simulink model "Load_Flow_Simulink"  (R2020b)
settings: Solver=FixedStepDiscrete  StartTime=0.0  StopTime=inf  FixedStep=0.001  RelTol=1e-3  EnableMultiTasking=on
InitFcn:
  | s1_define_network
  | s2_network_setup
  | s4_ybus2
  | 
  | %s3_ybus1
  | %s4_ybus2
  | 
  | 
  | %s5_dummy_load
  | 
  | %load('loadsDummy.mat')
values from neighbouring files (symbols this model uses):
  ABI = availableBusIndices    [Create_Ybus.m]
  Admittance = zeros(numBranch*3,5*3)    [s4_ybus2.m]    (also in s4_ybus3.m)
  BusFromTo = [busFrom busTo]    [s2_network_setup.m]
  busIDs = str2double(busNames)    [s1_define_network.m]
  busNames = [busNames(1:substationIndex-1); busNames(substationIndex+1:end);                busNames(substationIndex)]    [s1_define_network.m]    (also in s2_network_setup.m = int16(str2num(cell2mat(busNames))); s4_ybus3.m = int16(str2num(cell2mat(busNames))); s5_dummy_load.m = int16(str2num(cell2mat(busNames))))
  Ibase = Vbase/Zbase    [s1_define_network.m]
  LineCodes = [lineCodes;2]    [s1_define_network.m]    (also in s2_network_setup.m = zeros(37,1))
  loadsDummy = [600 600 2000 3000 100 100 100 0 0 0 0 0 ... (42 elements, 7x6)]    [loadsDummy.mat]    (also in s1_define_network.m = loadsIn)
  MBI = missingBusIndices    [Create_Ybus.m]    (also in s2_network_setup.m = 0)
  N = numBus-1    [Create_Ybus.m]
  noLoadQuantities = v2struct(v0mags,v0phases,v0,w,wCheck,w3phase)    [Compute_No_Load_Voltage.m]    (also in s2_network_setup.m = Compute_No_Load_Voltage(Y,Y_NS,N,                           )
  numBranch = length(lineBuses1)    [Create_Ybus.m]    (also in s1_define_network.m)
  numLines = 34    [s1_define_network.m]
  PNLI = phaseNodesLinIndices    [Create_Ybus.m]
  Sbase = 2500000    [s1_define_network.m]
  Y = Ynet(1:end-3,1:end-3)    [Create_Ybus.m]    (also in s2_network_setup.m = full(Y); s4_ybus3.m)
  Y_NS = Ynet(1:end-3,end-2:end)    [Create_Ybus.m]    (also in s2_network_setup.m = full(Y_NS); s4_ybus3.m)
undefined symbols (not defined in the file or in its folder): regulator
libraries: rtlab x1
Description:
  | Model of a simple control system for use iin training.
settings Model: Creator=Paul Baracos  LastModifiedBy=xjk374
settings DataIOCC: LimitDataPoints=on  SaveFormat=Array  SignalLoggingSaveFormat=ModelDataLogs  SaveOutput=off  SaveTime=off  ReturnWorkspaceOutputs=off  SignalLoggingName=sigsOut
settings OptimizationCC: BlockReduction=off  BooleanDataType=off  OptimizeBlockIOStorage=off  BufferReuse=off  ExpressionFolding=off  LocalBlockOutputs=off  InitFltsAndDblsToZero=on  LifeSpan=inf
settings DebuggingCC: SaveWithParameterizedLinksMsg=none  UnderspecifiedInitializationDetection=Classic  MergeDetectMultiDrivingBlocksExec=none  MultiTaskDSMMsg=warning  MultiTaskCondExecSysMsg=none  FcnCallInpInsideContextMsg=warning  SFUnexpectedBacktrackingDiag=warning  SFNoUnconditionalDefaultTransitionDiag=warning  SFExecutionAtInitializationDiag=none  ArithmeticOperatorsInVariantConditions=warning
settings HardwareCC: ProdBitPerPointer=32  ProdBitPerSizeT=32  ProdBitPerPtrDiffT=32  ProdLargestAtomicFloat=None  ProdIntDivRoundTo=Undefined  ProdEndianess=Unspecified  ProdWordSize=32  ProdHWDeviceType=32-bit Generic  TargetBitPerPointer=64  TargetBitPerSizeT=64  TargetBitPerPtrDiffT=64  TargetLongLongMode=on  TargetIntDivRoundTo=Zero  TargetEndianess=LittleEndian  TargetWordSize=64  TargetHWDeviceType=MATLAB Host  ProdEqTarget=off
settings ModelReferenceCC: PropagateSignalLabelsOutOfModel=off
settings SFSimCC: SimUseLocalCustomCode=off  CustomCodeUndefinedFunction=UseInterfaceOnly
settings RTWCC: RTWUseLocalCustomCode=off
settings CodeAppCC: StateflowObjectComments=on
settings GRTTargetCC: TargetFcnLib=ansi_tfl_tmw.mat  TargetLangStandard=C89/C90 (ANSI)  CombineOutputUpdateFcns=off  GRTInterface=on
settings ConfigComp: CovMetricSettings=dw  CovSaveCumulativeToWorkspaceVar=on  CovSaveSingleToWorkspaceVar=on  CovExternalEMLEnable=off

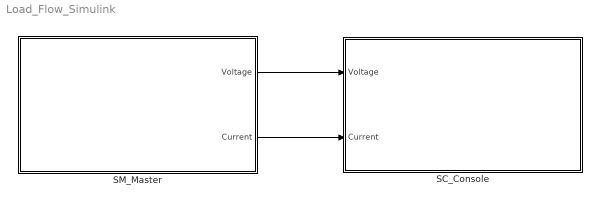
== system Load_Flow_Simulink ==
  SC_Console : Subsystem
  SM_Master : Subsystem
  wires:
  SM_Master/2(Current) -> SC_Console/2(Current)
  SM_Master/1(Voltage) -> SC_Console/1(Voltage)

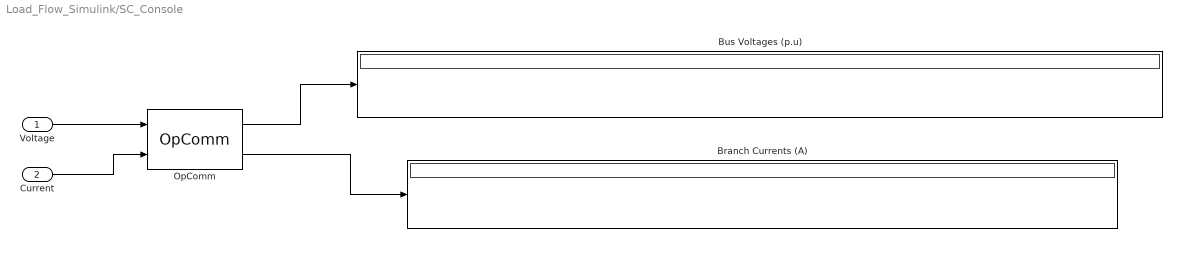
== system Load_Flow_Simulink/SC_Console ==
  Voltage : Inport
  Current : Inport  Port=2
  Branch Currents (A) : Display
  Bus Voltages (p.u) : Display
  OpComm : rtlab/OpComm  nbport=2  groupe_acq=1  subsys_rate=0  st=0  Synchronization=on  Interpolation=on  Threshold=1.0  Missed_Data=off  Sim_Time=off  Samples=off  dynSigOut=off  from_console=0  warning_done=off  writeOpCommFile=off  Offset=off
      settings: SourceProductName=RT-LAB
  wires:
  Voltage/1 -> OpComm/1
  Current/1 -> OpComm/2
  OpComm/1 -> Bus Voltages (p.u)/1
  OpComm/2 -> Branch Currents (A)/1

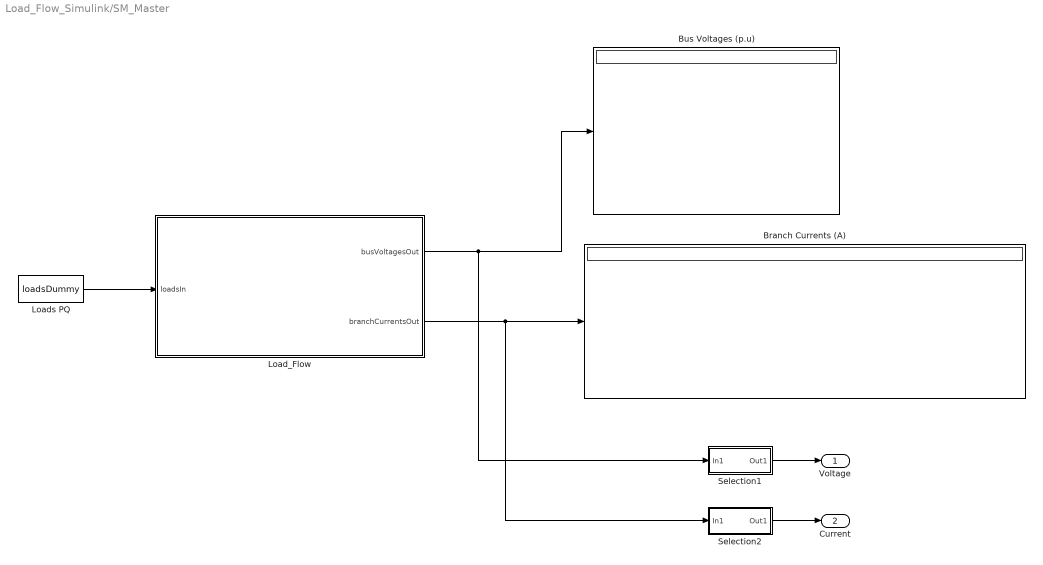
== system Load_Flow_Simulink/SM_Master ==
  Branch Currents (A) : Display
  Bus Voltages (p.u) : Display
  Load_Flow : MATLAB Function  TreatAsAtomicUnit=on
  Loads PQ : Constant  Value=loadsDummy
  Selection1 : Subsystem
  Selection2 : Subsystem
  Voltage : Outport
  Current : Outport  Port=2
  wires:
  Loads PQ/1 -> Load_Flow/1(loadsIn)
  Load_Flow/1(busVoltagesOut) -> Bus Voltages (p.u)/1, Selection1/1(In1)
  Load_Flow/2(branchCurrentsOut) -> Branch Currents (A)/1, Selection2/1(In1)
  Selection1/1(Out1) -> Voltage/1
  Selection2/1(Out1) -> Current/1

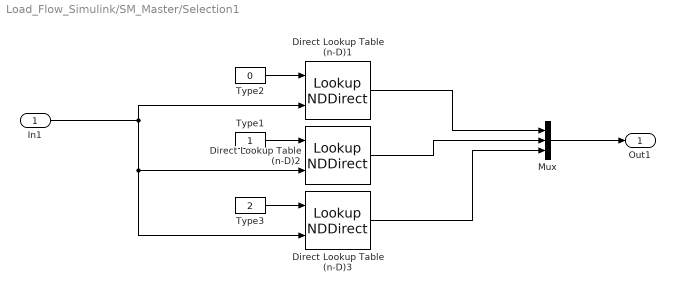
== system Load_Flow_Simulink/SM_Master/Selection1 ==
  In1 : Inport
  Direct Lookup Table (n-D)1 : LookupNDDirect  InputsSelectThisObjectFromTable=Vector  TableIsInput=on
  Direct Lookup Table (n-D)2 : LookupNDDirect  InputsSelectThisObjectFromTable=Vector  TableIsInput=on
  Direct Lookup Table (n-D)3 : LookupNDDirect  InputsSelectThisObjectFromTable=Vector  TableIsInput=on
  Mux : Mux  Inputs=3
  Type1 : Constant
  Type2 : Constant  Value=0
  Type3 : Constant  Value=2
  Out1 : Outport
  wires:
  Direct Lookup Table (n-D)2/1 -> Mux/2
  Type3/1 -> Direct Lookup Table (n-D)3/1
  Type1/1 -> Direct Lookup Table (n-D)2/1
  Mux/1 -> Out1/1
  In1/1 -> Direct Lookup Table (n-D)3/2, Direct Lookup Table (n-D)2/2, Direct Lookup Table (n-D)1/2
  Type2/1 -> Direct Lookup Table (n-D)1/1
  Direct Lookup Table (n-D)3/1 -> Mux/3
  Direct Lookup Table (n-D)1/1 -> Mux/1

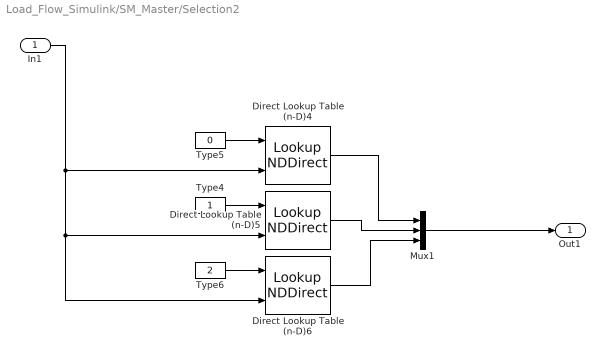
== system Load_Flow_Simulink/SM_Master/Selection2 ==
  In1 : Inport
  Direct Lookup Table (n-D)4 : LookupNDDirect  InputsSelectThisObjectFromTable=Vector  TableIsInput=on
  Direct Lookup Table (n-D)5 : LookupNDDirect  InputsSelectThisObjectFromTable=Vector  TableIsInput=on
  Direct Lookup Table (n-D)6 : LookupNDDirect  InputsSelectThisObjectFromTable=Vector  TableIsInput=on
  Mux1 : Mux  Inputs=3
  Type4 : Constant
  Type5 : Constant  Value=0
  Type6 : Constant  Value=2
  Out1 : Outport
  wires:
  Direct Lookup Table (n-D)4/1 -> Mux1/1
  Direct Lookup Table (n-D)5/1 -> Mux1/2
  In1/1 -> Direct Lookup Table (n-D)4/2, Direct Lookup Table (n-D)5/2, Direct Lookup Table (n-D)6/2
  Direct Lookup Table (n-D)6/1 -> Mux1/3
  Type5/1 -> Direct Lookup Table (n-D)4/1
  Type4/1 -> Direct Lookup Table (n-D)5/1
  Mux1/1 -> Out1/1
  Type6/1 -> Direct Lookup Table (n-D)6/1

== matlab function Load_Flow_Simulink/SM_Master/Load_Flow ==
  data: N parameter; Y parameter; Y_NS parameter; ABI parameter; MBI parameter; busIDs parameter; regulator parameter; busVoltagesOut output size=[numBus,3] [-inf..inf]; branchCurrentsOut output size=[numLines,3] [-inf..inf]; noLoadQuantities parameter; numBranch parameter; BusFromTo parameter; LineCodes parameter; loadsIn input; Admittance parameter; Ibase parameter; busNames parameter; Sbase parameter; PNLI parameter; numLines parameter
function [busVoltagesOut,branchCurrentsOut]= load_flow(N, Y, Y_NS, ABI, MBI, busIDs,regulator, noLoadQuantities,...
    numBranch,BusFromTo, LineCodes, loadsIn,... % R
    Admittance,... % K
    Ibase,... % H
    busNames,Sbase,...
PNLI, numLines)


%% LOAD_FLOW Run load flow in real-time
%   This simulink function should take the current load demand, then output
%   the branch currents (in CYME report format) for processing by the
%   optimization
% Need ro run before: network_setup.m, setupYbus_1.m, setupYbus_22.m
% There are 4 hardsets for each network: 1 in s1, 2 below (numBus, mode), 1
% parameter (busVoltagesOut)

% Hardset numBus to fix variable output error.
numBus = 37;

% % mode 0=IEEE 1=CYME
% mode = 0;

Y_NS = sparse(Y_NS);
Y = sparse(Y);

busNamesCell = cell(numBus,1);
for i=1:numBus
    busNamesCell{i} = sprintf('%03i',busNames(i));
end

% before computing branch currents, remove non-line elements
% only first 34 rows are lines
if numBus == 37
    BusFromToLines = BusFromTo(1:34,:);
    numBranch = 34;
    
elseif numBus ==9
    BusFromToLines = BusFromTo;
end



branchCurrents = complex(zeros(numBranch,3));
branchCurrentsOut = zeros(numBranch,3);

busVoltages = complex(zeros(numBus,3));
busVoltagesOut = zeros(numBus,3);
busVoltagesOutA = zeros(numBus,1);
v = zeros(numBus,1);
v3phase = zeros(numBus,1);

% FUNCTION 3
% input 'loads' is now a (numLoad,6) matrix
% must pre-define loadBuses and loadTypes

% IEEE37BUS
if numBus == 37
    loadBuses = [701;712;713;714;718;720;722;724;725;727;728;729;730;731;732;733;734;735;736;737;738;740;741;742;744];
    loadTypes = {'D-PQ';'D-PQ';'D-PQ';'D-I';'D-Z';'D-PQ';'D-I';'D-Z';'D-PQ';'D-PQ';'D-PQ';'D-I';'D-Z';'D-Z';'D-PQ';'D-I';'D-PQ';'D-PQ';'D-Z';'D-I';'D-PQ';'D-PQ';'D-I';'D-Z';'D-PQ'};
    [ sL_load,iL_load,yL_load,ePage,gMat,cMat,YL] = Setup_Loads_v2(loadBuses,loadTypes,loadsIn,N,busNamesCell,Sbase,noLoadQuantities,ABI,PNLI);
% loadQuantities = Setup_Loads(loads,N,busNames,Sbase,noLoadQuantities,ABI,PNLI);
end

% 9BUS
if numBus == 9
    loadBuses = [200,201,203,202,300,301,302]';
%     loadTypes = {'D-Z';'D-Z';'D-Z';'D-Z';'D-Z';'D-Z';'D-Z'};
    loadTypes = {'Y-Z';'Y-Z';'Y-Z';'Y-Z';'Y-Z';'Y-Z';'Y-Z'};
    [ sL_load,iL_load,yL_load,ePage,gMat,cMat,YL] = Setup_Loads_simulink(loadBuses,loadTypes,loadsIn,N,busNamesCell,Sbase,noLoadQuantities,ABI,PNLI);
end

% FUNCTION 4
ZBusResults = Perform_ZBus(noLoadQuantities,sL_load,iL_load,yL_load,ePage,gMat,cMat,YL,N,Y,Y_NS,ABI,MBI);

% FUNCTION 5

% IEEE with Regulators Mode
% if mode == 0
%     regulatorTypes = 'non-ideal';
%     busVoltages = Obtain_Voltages(busIDs,noLoadQuantities,N,ZBusResults,...
%                   regulatorTypes,regulator);
%     busVoltagesOut = [abs(busVoltages) ];
% end

% regulatorTypes = 'non-ideal';

if numBus == 37
    v = ZBusResults.v;
    v3phase=reshape(v,3,N+1).';
    v3phase = v3phase(1:end-1,:); % cutoff last row
    busVoltages = abs(v3phase);                       
    busVoltagesOut(:) = abs(v3phase);
end


if numBus == 9
    v = ZBusResults.v;
    v3phase=reshape(v,3,N+1).';
    busVoltages = abs(v3phase);                       
    busVoltagesOut(:) = abs(v3phase);
end

busVoltagesOutA = busVoltagesOut(:,1);

% FUNCTION 6 - KRISHNA BRANCH CURRENT         

% IEEE37BrCurrents = setupYbusIEEE37new('ideal',1e-6); % Run this before-hand
% iBrcurrents = cell2mat(computebranchcurrnets(IEEE37,IEEE37BrCurrents));
% IBrcurrents_pu = reshape(iBrcurrents,3,length(IEEE37BrCurrents.Branch.Numbers)).';



[branchCurrents] = Compute_Branch_Currents_alt(...
    numBranch,... % DistributionNetwork
    BusFromToLines,...
    LineCodes,...
    busIDs,...
    v3phase,...   % ZBusSolution
    Admittance);

branchCurrentsOut(:,:) = abs(reshape(branchCurrents,3,numBranch).');

branchCurrentsOut = branchCurrentsOut*Ibase;

% branchCurrentsOutA = branchCurrentsOut(:,1);

% branchCurrents = zeros(numBranch,3);
% busVoltagesOut = zeros(numBus,3);

% branchCurrents = IBrcurrents_pu;

% busVoltages = u;
% branchCurrents = 7;
